simulink model "dommotorSimscape"  (R2016a)
settings: Solver=ode23t  StartTime=0.0  StopTime=10  RelTol=1e-3  AbsTol=1e-3
libraries: fl_lib x13, nesl_utility x3, pe_lib x1
settings Model: Creator=mmdclm  LastModifiedBy=Lara
settings GRTTargetCC: GeneratePreprocessorConditionals=Use local settings
settings SimscapeCC: SimscapeLogType=all  SimscapeLogDataHistory=10000

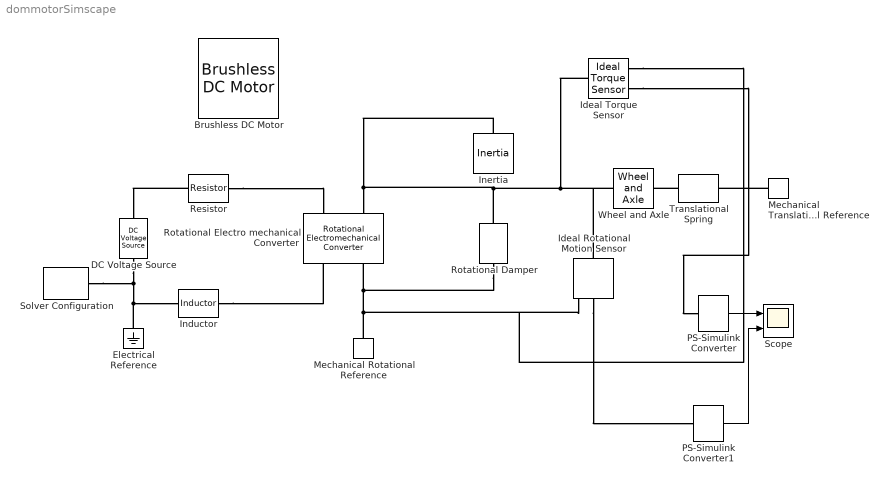
== system dommotorSimscape ==
  Brushless DC Motor : pe_lib/Machines/Permanent Magnet Rotor/Brushless DC Motor  rotor_param=1  pm_flux_linkage=0.03 Wb  theta_constant=pi / 12 rad  emf_max=9.6 V  DphiDtheta_tab=[0.0, -0.1528, -0.1528, 0.1528, 0.1528, 0.0] Wb/rad  back_emf_tab=[0.0, 9.6, 9.6, -9.6, -9.6, 0.0] V  rotor_angle_tab=[0.0, 7.5, 22.5, 37.5, 52.5, 60.0] deg  w_meas=600 rpm  nPolePairs=6  stator_param=1  Ld=0.00022 H  Lq=0.00022 H  L0=0.00016 H  Ls=0.0002 H  Lm=0 H  Ms=0.00002 H  Rs=0.013 Ohm  initial_currents=[0.0, 0.0, 0.0] A  axes_param=2  angular_position0=0 deg
  DC Voltage Source : fl_lib/Electrical/Electrical Sources/DC Voltage Source  v0=360 V
  Electrical Reference : fl_lib/Electrical/Electrical Elements/Electrical Reference
  Ideal Rotational Motion Sensor : fl_lib/Mechanical/Mechanical Sensors/Ideal Rotational Motion Sensor  offset=0 rad
  Ideal Torque Sensor : fl_lib/Mechanical/Mechanical Sensors/Ideal Torque Sensor
  Inductor : fl_lib/Electrical/Electrical Elements/Inductor  l=18.7e-3 H  r=0 Ohm  g=1e-9 1/Ohm  i_specify=off  i_priority=None  i=0 A  v_specify=off  v_priority=None  v=0 V  i_L_specify=off  i_L_priority=High  i_L=0 A
  Inertia : fl_lib/Mechanical/Rotational Elements/Inertia  inertia=270 g*cm^2  w_specify=off  w_priority=High  w=0 rad/s  t_specify=off  t_priority=None  t=0 N*m
  Mechanical Rotational Reference : fl_lib/Mechanical/Rotational Elements/Mechanical Rotational Reference
  Mechanical Translational Reference : fl_lib/Mechanical/Translational Elements/Mechanical Translational Reference
  PS-Simulink Converter : nesl_utility/PS-Simulink Converter  PhysicalDomain=network_engine_domain  SubClassName=ps_output  LeftPortType=input  RightPortType=output  PseudoPeriodic=off  Frequencies=[]  Unit=N*m  AffineConversion=off
  PS-Simulink Converter1 : nesl_utility/PS-Simulink Converter  PhysicalDomain=network_engine_domain  SubClassName=ps_output  LeftPortType=input  RightPortType=output  PseudoPeriodic=off  Frequencies=[]  Unit=rad/s  AffineConversion=off
  Resistor : fl_lib/Electrical/Electrical Elements/Resistor  R=9.02 Ohm  i_specify=off  i_priority=None  i=0 A  v_specify=off  v_priority=None  v=0 V
  Rotational Electro mechanical Converter : fl_lib/Electrical/Electrical Elements/Rotational Electromechanical Converter  K=0.5 V/(rad/s)  i_specify=on  i_priority=None  i=0 A  v_specify=on  v_priority=None  v=0 V  t_specify=on  t_priority=None  t=0 N*m  w_specify=on  w_priority=None  w=0 rad/s
  Rotational Damper : fl_lib/Mechanical/Rotational Elements/Rotational Damper  D=0.007 N*m/(rad/s)  w_specify=off  w_priority=None  w=0 rad/s  t_specify=off  t_priority=None  t=0 N*m
  Scope : Scope  NumInputPorts=2
  Solver Configuration : nesl_utility/Solver Configuration  PhysicalDomain=network_engine_domain  SubClassName=solver  LeftPortType=input  RightPortType=generic  Accelerate=off  Tones=[]  Harmonics=[]  SimulateNoise=off  Profile=off  UseLocalSampling=off  EnableSwitchedLinearOptims=on  FrequencyDomain=off  UseCCode=off  RelTol=0.001  AbsTol=1e-06  MinStep=1e-09  ToWorkspace=off  RevertToSquareIcSolve=off  NumHomotopyIterations=100  PhasorMode=off  PhasorModeNumHarmonics=1  OverrideAbsTol=off  DoDC=off  ResidualTolerance=1e-09  UseLocalSolver=off  LocalSolverChoice=NE_BACKWARD_EULER_ADVANCER  LocalSolverSampleTime=0.001  DoFixedCost=off  MaxNonlinIter=3  MaxModeIter=2  LinearAlgebra=Sparse  DelaysMemoryBudget=1024  AutomaticFiltering=on  FilteringTimeConstant=0.001
  Translational Spring : fl_lib/Mechanical/Translational Elements/Translational Spring  spr_rate=1000 N/m  v_specify=off  v_priority=None  v=0 m/s  f_specify=off  f_priority=None  f=0 N  x_specify=off  x_priority=High  x=0 m
  Wheel and Axle : fl_lib/Mechanical/Mechanisms/Wheel and Axle  R=0.05 m  or=1  t_specify=off  t_priority=None  t=0 N*m  f_specify=off  f_priority=None  f=0 N
  wires:
  PS-Simulink Converter/1 -> Scope/1
  PS-Simulink Converter1/1 -> Scope/2
  connections:
  Resistor/LConn1 -- DC Voltage Source/LConn1
  Resistor/RConn1 -- Rotational Electro mechanical Converter/LConn1
  DC Voltage Source/RConn1 -- Solver Configuration/RConn1 -- Electrical Reference/LConn1 -- Inductor/LConn1
  Inductor/RConn1 -- Rotational Electro mechanical Converter/RConn1
  Mechanical Rotational Reference/LConn1 -- Ideal Torque Sensor/RConn1 -- Ideal Rotational Motion Sensor/RConn1 -- Rotational Damper/RConn1 -- Rotational Electro mechanical Converter/RConn2
  Inertia/LConn1 -- Ideal Torque Sensor/LConn1 -- Wheel and Axle/LConn1 -- Ideal Rotational Motion Sensor/LConn1 -- Rotational Damper/LConn1 -- Rotational Electro mechanical Converter/LConn2
  Translational Spring/LConn1 -- Wheel and Axle/RConn1
  Mechanical Translational Reference/LConn1 -- Translational Spring/RConn1
  Ideal Rotational Motion Sensor/RConn2 -- PS-Simulink Converter1/LConn1
  Ideal Torque Sensor/RConn2 -- PS-Simulink Converter/LConn1
